simulink model "abb_op_space_hybrid"  (R2023b)
settings: Solver=ode45  StartTime=0.0  StopTime=inf  RelTol=1e-3
undefined symbols (not defined in the file): abb_eom_solution, abbRobot, control_op_space_hybrid, hamiltonian_fun_solution, I_Je_fun_solution, I_r_IE_fun_solution
libraries: simulink x4
settings Model: Creator=dario  LastModifiedBy=slin
settings SolverCC: AlgebraicLoopSolver=TrustRegion
settings DataIOCC: LimitDataPoints=on  SaveFormat=Array  ReturnWorkspaceOutputs=off
settings OptimizationCC: BlockReduction=off  BooleanDataType=off  LifeSpan=inf
settings DebuggingCC: SaveWithParameterizedLinksMsg=none  UnderspecifiedInitializationDetection=Classic  MergeDetectMultiDrivingBlocksExec=none  SignalResolutionControl=TryResolveAllWithWarning  FcnCallInpInsideContextMsg=warning  UnconnectedInputMsg=warning  UnconnectedOutputMsg=warning  UnconnectedLineMsg=warning  SFUnexpectedBacktrackingDiag=warning  SFNoUnconditionalDefaultTransitionDiag=warning  ArithmeticOperatorsInVariantConditions=warning
settings HardwareCC: ProdBitPerPointer=32  ProdBitPerSizeT=32  ProdBitPerPtrDiffT=32  ProdLargestAtomicFloat=None  ProdIntDivRoundTo=Undefined  ProdEndianess=Unspecified  ProdWordSize=32  ProdHWDeviceType=32-bit Generic  TargetUnknown=on
settings ModelReferenceCC: EnableRefExpFcnMdlSchedulingChecks=on  PropagateSignalLabelsOutOfModel=off
settings SFSimCC: SimUseLocalCustomCode=off  CustomCodeUndefinedFunction=UseInterfaceOnly
settings RTWCC: RTWUseLocalCustomCode=off
settings CodeAppCC: StateflowObjectComments=on
settings GRTTargetCC: TargetLangStandard=C89/C90 (ANSI)
settings ConfigComp: CovMetricSettings=dw  CovSaveCumulativeToWorkspaceVar=on  CovSaveSingleToWorkspaceVar=on  CovExternalEMLEnable=off

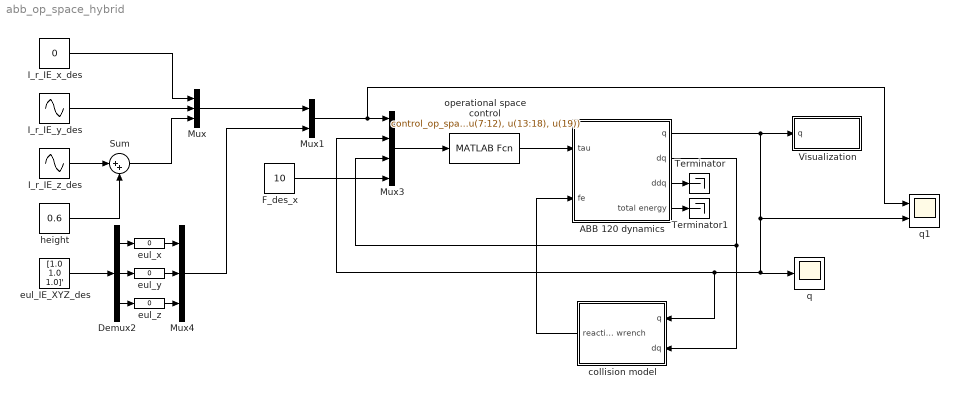
== system abb_op_space_hybrid ==
  ABB 120 dynamics : Subsystem  mask{Ts=0.01, F=[0.1 0.1 0.1 0.1 0.1 0.1]', phi0=[0 -pi/4 pi/4 0 0 0]', dphi0=[0 0 0 0 0 0]', enable_g=on, enable_f=off}
      mask prompts: Ts "Sample time"; F "Viscous friction (6x1)"; phi0 "Initial joint positions"; dphi0 "Initial joint velocities"; enable_g "Enable gravity"; enable_f "Enable friction"
  Demux2 : Demux  Outputs=3
  F_des_x : Constant  Value=10
  I_r_IE_x_des : Constant  Value=0
  I_r_IE_y_des : Sin  Amplitude=0.1  Frequency=2*pi*0.2  Phase=pi/2  SampleTime=0
  I_r_IE_z_des : Sin  Amplitude=0.1  Frequency=2*pi*0.2  SampleTime=0
  Mux : Mux  Inputs=3
  Mux1 : Mux  Inputs=2
  Mux3 : Mux
  Mux4 : Mux  Inputs=3
  Sum : Sum  Inputs=|++
  Terminator : Terminator
  Terminator1 : Terminator
  Visualization : Subsystem
  collision model : Subsystem  mask{x_wall=0.4}
      mask prompts: x_wall "The position of the wall on the x axis"
  eul_IE_XYZ_des : Constant  Value=[1.0 1.0 1.0]'
  eul_x : simulink/Math Operations/Slider Gain  gain=0  low=-2  high=2
  eul_y : simulink/Math Operations/Slider Gain  gain=0  low=-2  high=2
  eul_z : simulink/Math Operations/Slider Gain  gain=0  low=-2  high=2
  height : Constant  Value=0.6
  operational space control : MATLABFcn  MATLABFcn=control_op_space_hybrid( u(1:3), u(4:6), u(7:12), u(13:18), u(19))  OutputDimensions=[6,1]  Output1D=off
  q : Scope
  q1 : Scope  NumInputPorts=2
  wires:
  ABB 120 dynamics/1(q) -> Mux3/2, collision model/1(q), q/1, q1/2, Visualization/1(q)
  Mux3/1 -> operational space control/1
  ABB 120 dynamics/2(dq) -> collision model/2(dq), Mux3/3
  operational space control/1 -> ABB 120 dynamics/1(tau)
  F_des_x/1 -> Mux3/4
  collision model/1(reaction wrench) -> ABB 120 dynamics/2(fe)
  Mux/1 -> Mux1/1
  Mux1/1 -> q1/1, Mux3/1
  I_r_IE_y_des/1 -> Mux/2
  I_r_IE_x_des/1 -> Mux/1
  I_r_IE_z_des/1 -> Sum/1
  Sum/1 -> Mux/3
  height/1 -> Sum/2
  ABB 120 dynamics/3(ddq) -> Terminator/1
  ABB 120 dynamics/4(total energy) -> Terminator1/1
  Demux2/1 -> eul_x/1
  Demux2/2 -> eul_y/1
  eul_z/1 -> Mux4/3
  eul_y/1 -> Mux4/2
  eul_x/1 -> Mux4/1
  Demux2/3 -> eul_z/1
  eul_IE_XYZ_des/1 -> Demux2/1
  Mux4/1 -> Mux1/2

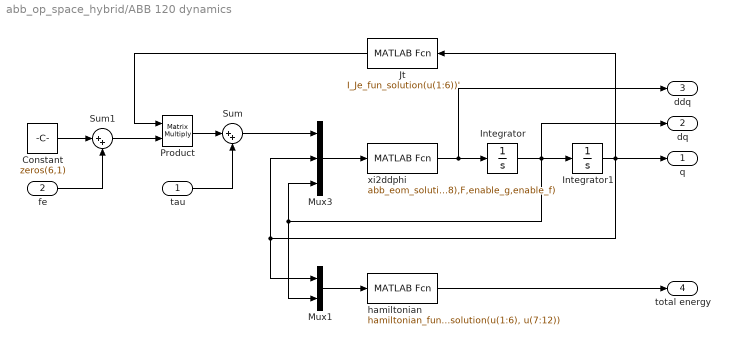
== system abb_op_space_hybrid/ABB 120 dynamics ==
  tau : Inport
  fe : Inport  Port=2
  Constant : Constant  Value=zeros(6,1)
  Integrator : Integrator  InitialCondition=dphi0
  Integrator1 : Integrator  InitialCondition=phi0
  Jt : MATLABFcn  MATLABFcn=I_Je_fun_solution(u(1:6))'  OutputDimensions=[6,6]  OutputSignalType=real  Output1D=off
  Mux1 : Mux  Inputs=2
  Mux3 : Mux  Inputs=3
  Product : Product  Multiplication=Matrix(*)
  Sum : Sum  Inputs=|++
  Sum1 : Sum  Inputs=|++
  hamiltonian : MATLABFcn  MATLABFcn=hamiltonian_fun_solution(u(1:6), u(7:12))  OutputDimensions=[1,1]  Output1D=off
  xi2ddphi : MATLABFcn  MATLABFcn=abb_eom_solution(u(1:6), u(7:12), u(13:18),F,enable_g,enable_f)  OutputDimensions=[6,1]  Output1D=off
  q : Outport
  dq : Outport  Port=2
  ddq : Outport  Port=3
  total energy : Outport  Port=4
  wires:
  Integrator/1 -> Mux1/2, Mux3/3, dq/1, Integrator1/1
  tau/1 -> Sum/2
  Integrator1/1 -> Jt/1, Mux1/1, Mux3/2, q/1
  Mux3/1 -> xi2ddphi/1
  xi2ddphi/1 -> ddq/1, Integrator/1
  Mux1/1 -> hamiltonian/1
  hamiltonian/1 -> total energy/1
  Jt/1 -> Product/1
  Product/1 -> Sum/1
  Sum/1 -> Mux3/1
  Constant/1 -> Sum1/1
  fe/1 -> Sum1/2
  Sum1/1 -> Product/2

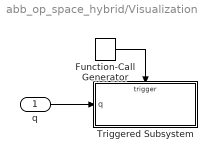
== system abb_op_space_hybrid/Visualization ==
  q : Inport
  Function-Call Generator : simulink/Ports & Subsystems/Function-Call Generator  sample_time=0.05  numberOfIterations=1  DisallowWideOutput=off
  Triggered Subsystem : Subsystem  TreatAsAtomicUnit=on
  wires:
  Function-Call Generator/1 -> Triggered Subsystem/Trigger
  q/1 -> Triggered Subsystem/1(q)

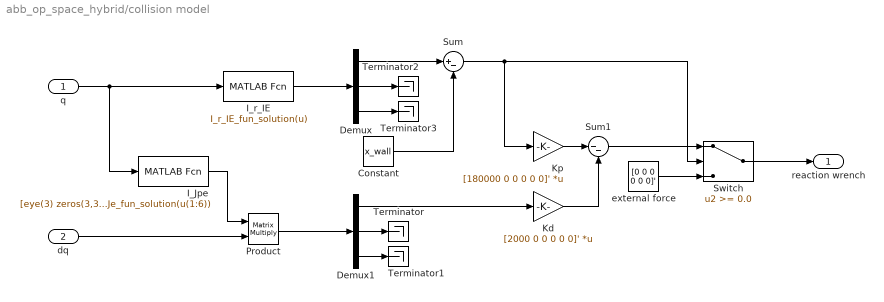
== system abb_op_space_hybrid/collision model ==
  q : Inport
  dq : Inport  Port=2
  Constant : Constant  Value=x_wall
  Demux : Demux  Outputs=3
  Demux1 : Demux  Outputs=3
  I_Jpe : MATLABFcn  MATLABFcn=[eye(3) zeros(3,3)] * I_Je_fun_solution(u(1:6))  OutputDimensions=[3,6]  Output1D=off
  I_r_IE : MATLABFcn  MATLABFcn=I_r_IE_fun_solution(u)  OutputDimensions=[3,1]  Output1D=off
  "Kd " : Gain  Gain=[2000 0 0 0 0 0]'  Multiplication=Matrix(K*u)
  Kp : Gain  Gain=[180000 0 0 0 0 0]'  Multiplication=Matrix(K*u)
  Product : Product  Multiplication=Matrix(*)
  Sum : Sum  Inputs=|+-
  Sum1 : Sum  Inputs=|--
  Switch : Switch  Threshold=0.0  SaturateOnIntegerOverflow=off  InputSameDT=off
  Terminator{,1..3} (4 alike) : Terminator
  external force : Constant  Value=[0 0 0 0 0 0]'
  reaction wrench : Outport
  wires:
  Sum1/1 -> Switch/1
  Constant/1 -> Sum/2
  dq/1 -> Product/2
  Kp/1 -> Sum1/1
  external force/1 -> Switch/3
  Demux/2 -> Terminator2/1
  Demux1/3 -> Terminator1/1
  Demux/1 -> Sum/1
  Sum/1 -> Kp/1, Switch/2
  Demux1/1 -> "Kd "/1
  I_r_IE/1 -> Demux/1
  Demux1/2 -> Terminator/1
  q/1 -> I_r_IE/1, I_Jpe/1
  Demux/3 -> Terminator3/1
  I_Jpe/1 -> Product/1
  Product/1 -> Demux1/1
  Switch/1 -> reaction wrench/1
  "Kd "/1 -> Sum1/2

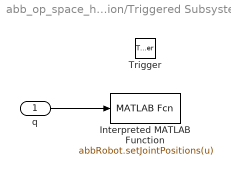
== system abb_op_space_hybrid/Visualization/Triggered Subsystem ==
  q : Inport
  Trigger : TriggerPort  TriggerType=function-call  VariantControl=Variant
  Interpreted MATLAB Function : MATLABFcn  MATLABFcn=abbRobot.setJointPositions(u)  OutputDimensions=0
  wires:
  q/1 -> Interpreted MATLAB Function/1
